simulink model "velpos_controller"  (R2018a)
settings: Solver=FixedStepDiscrete  StartTime=0.0  StopTime=10.0  FixedStep=0.01  RelTol=1e-3
libraries: simulink_extras x2, discretizing x2, simulink x1
settings Model: Creator=Matteo  LastModifiedBy=Matteo
settings OptimizationCC: DefaultParameterBehavior=Inlined  EnhancedBackFolding=on  PassReuseOutputArgsAs=Individual arguments  OptimizeBlockOrder=speed  DifferentSizesBufferReuse=on
settings DebuggingCC: ParameterTunabilityLossMsg=error
settings SFSimCC: MATLABDynamicMemAlloc=off
settings RTWCC: SystemTargetFile=ert.tlc  TemplateMakefile=ert_default_tmf  GenerateReport=on  IncludeHyperlinkInReport=on  LaunchReport=on  GenerateTraceInfo=on  GenerateTraceReport=on  GenerateTraceReportSl=on  GenerateTraceReportSf=on  GenerateTraceReportEml=on
settings CodeAppCC: ForceParamTrailComments=on  IgnoreCustomStorageClasses=off  OperatorAnnotations=on  SimulinkDataObjDesc=on  SFDataObjDesc=on  InsertBlockDesc=on
settings ERTTargetCC: TargetLangStandard=C99 (ISO)  GenerateSampleERTMain=on  InlinedParameterPlacement=NonHierarchical  ERTCustomFileTemplate=example_file_process.tlc

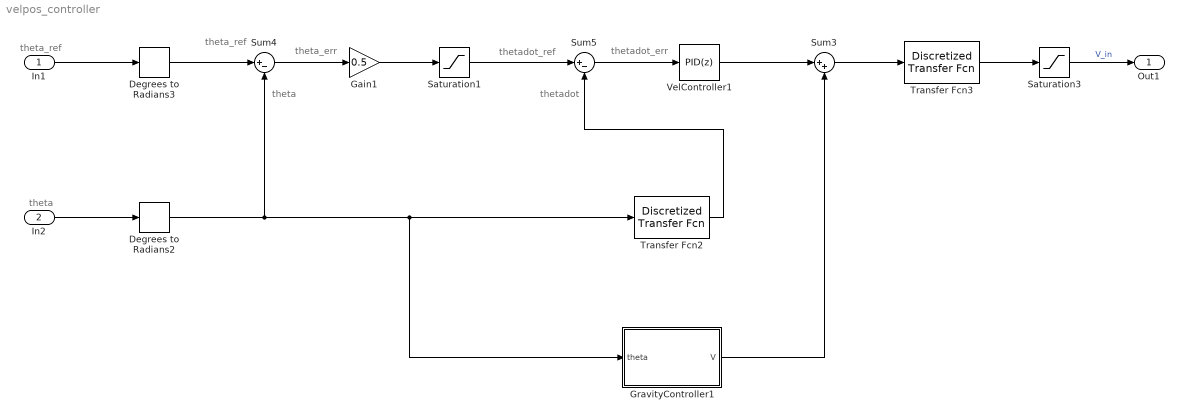
== system velpos_controller ==
  note: theta
  note: theta_ref
  note: theta
  note: thetadot_err
  note: thetadot
  note: thetadot_ref
  note: theta_err
  note: theta_ref
  In1 : Inport
  In2 : Inport  Port=2
  Degrees to Radians2 : simulink_extras/Transformations/Degrees to Radians
  Degrees to Radians3 : simulink_extras/Transformations/Degrees to Radians
  Gain1 : Gain  Gain=0.5
  GravityController1 : Subsystem  mask{pwm90=200*24/4095, M=0.46700000, d=0.21666702, g=9.81, kt=0.08444, Kp=1.5, Kd=0, Ki=10}
      mask prompts: pwm90 "pwm at 90deg"; M "Mass"; d "distance CoM"; g "gravity accel"; kt "torque const"; Kp "proportional gain"; Kd "derivative gain"; Ki "integral gain"
  Saturation1 : Saturate  UpperLimit=0.1  LowerLimit=-0.1
  Saturation3 : Saturate  UpperLimit=10  LowerLimit=-10
  Sum3 : Sum  Inputs=|++
  Sum4 : Sum  Inputs=|+-
  Sum5 : Sum  Inputs=|+-
  Transfer Fcn2 : discretizing/Discretized Transfer Fcn  Numerator=[1 0]  Denominator=[1/25 1]  AbsTol=auto  SampleTime=0.01  method=zoh  Wc=1
  Transfer Fcn3 : discretizing/Discretized Transfer Fcn  Numerator=[1 ]  Denominator=[1/5 1]  AbsTol=auto  SampleTime=0.01  method=zoh  Wc=1
  VelController1 : simulink/Continuous/PID Controller  Controller=PID  TimeDomain=Discrete-time  SampleTime=-1  IntegratorMethod=Trapezoidal  FilterMethod=Trapezoidal  Form=Parallel  UseFilter=on  ControllerParametersSource=internal  P=5  I=0.7  D=0  N=182  InitialConditionSource=internal  InitialConditionForIntegrator=0  InitialConditionForFilter=0  ExternalReset=none  LimitOutput=off  UpperSaturationLimit=inf  LowerSaturationLimit=-inf  LinearizeAsGain=off  AntiWindupMode=none  Kb=1  TrackingMode=off  Kt=1  PParamMin=[]  PParamMax=[]  IParamMin=[]  IParamMax=[]  DParamMin=[]  DParamMax=[]  NParamMin=[]  NParamMax=[]  KbParamMin=[]  KbParamMax=[]  KtParamMin=[]  KtParamMax=[]  POutMin=[]  POutMax=[]  IOutMin=[]  IOutMax=[]  DOutMin=[]  DOutMax=[]  NOutMin=[]  NOutMax=[]  KbOutMin=[]  KbOutMax=[]  KtOutMin=[]  KtOutMax=[]  IntegratorOutMin=[]  IntegratorOutMax=[]  FilterOutMin=[]  FilterOutMax=[]  SumOutMin=[]  SumOutMax=[]  SumI1OutMin=[]  SumI1OutMax=[]  SumI2OutMin=[]  SumI2OutMax=[]  SumI3OutMin=[]  SumI3OutMax=[]  SumDOutMin=[]  SumDOutMax=[]  SaturationOutMin=[]  SaturationOutMax=[]  IntegratorContinuousStateAttributes=''  IntegratorStateMustResolveToSignalObject=off  IntegratorRTWStateStorageClass=Auto  FilterContinuousStateAttributes=''  FilterStateMustResolveToSignalObject=off  FilterRTWStateStorageClass=Auto  DifferentiatorICPrevScaledInput=0  DifferentiatorOutMin=[]  DifferentiatorOutMax=[]  FilterDiffOutCoefMin=[]  FilterDiffOutCoefMax=[]  SumDenOutMin=[]  SumDenOutMax=[]  SumNumOutMin=[]  SumNumOutMax=[]  ReciprocalOutMin=[]  ReciprocalOutMax=[]  DivideOutMin=[]  DivideOutMax=[]  TunerSelectOption=Transfer Function Based (PID Tuner App)
  Out1 : Outport
  wires:
  Degrees to Radians2/1 -> Sum4/2, Transfer Fcn2/1, GravityController1/1(theta)
  Sum5/1 -> VelController1/1
  Sum4/1 -> Gain1/1
  Transfer Fcn2/1 -> Sum5/2
  Transfer Fcn3/1 -> Saturation3/1
  VelController1/1 -> Sum3/1
  Sum3/1 -> Transfer Fcn3/1
  GravityController1/1(V) -> Sum3/2
  Degrees to Radians3/1 -> Sum4/1
  In1/1 -> Degrees to Radians3/1
  In2/1 -> Degrees to Radians2/1
  Saturation3/1 -> Out1/1  "V_in"
  Saturation1/1 -> Sum5/1
  Gain1/1 -> Saturation1/1

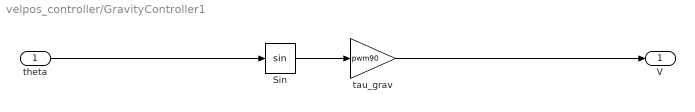
== system velpos_controller/GravityController1 ==
  theta : Inport
  Sin : Trigonometry
  tau_grav : Gain  Gain=pwm90
  V : Outport
  wires:
  Sin/1 -> tau_grav/1
  theta/1 -> Sin/1
  tau_grav/1 -> V/1
